simulink model "untitled"  (Simulink 7.5)
settings: Solver=ode45  StartTime=0.0  StopTime=5  RelTol=1e-3
libraries: simulink x1
settings Model: Creator=Anonymos  LastModifiedBy=Anonymos

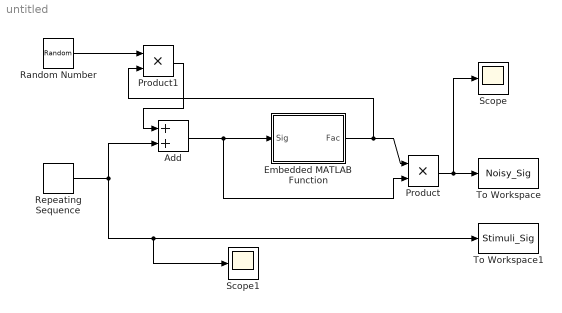
== system untitled ==
  Add : Sum  OutDataType=fixdt(1, 16)  OutScaling=2^-10
  Embedded MATLAB Function : Stateflow chart  TreatAsAtomicUnit=on
  Product : Product  OutDataType=fixdt(1, 16)  OutScaling=2^0  RndMeth=Zero
  Product1 : Product  OutDataType=fixdt(1, 16)  OutScaling=2^0  RndMeth=Zero
  Random Number : RandomNumber  Variance=0.0003132  Seed=234234  SampleTime=0.05
  Repeating Sequence : simulink/Sources/Repeating Sequence  SystemSampleTime=-1  rep_seq_t=[0 2]  rep_seq_y=[0 2]
  Scope : Scope
  Scope1 : Scope
  To Workspace : ToWorkspace  VariableName=Noisy_Sig  SampleTime=-1  SaveFormat=Array
  To Workspace1 : ToWorkspace  VariableName=Stimuli_Sig  SampleTime=-1  SaveFormat=Array
  wires:
  Repeating Sequence/1 -> Add/2, To Workspace1/1, Scope1/1
  Add/1 -> Embedded MATLAB Function/1(Sig), Product/2
  Embedded MATLAB Function/1(Fac) -> Product/1, Product1/2
  Product/1 -> To Workspace/1, Scope/1
  Random Number/1 -> Product1/1
  Product1/1 -> Add/1

== matlab function Embedded MATLAB Function ==
  data: Sig input double; Fac output double
function Fac = fcn(Sig)
%#eml

Fac=Sig/0.2;
